simulink model "RobotModel8"  (R2025b)
settings: Solver=VariableStepAuto  StartTime=0.0  StopTime=150  RelTol=0.01  AbsTol=0.01  EnableMultiTasking=on
values from neighbouring files (symbols this model uses):
  waypoints = [R*cos(theta)+5, R*sin(theta)]    [init_waypoints.m]
undefined symbols (not defined in the file or in its folder): X, Y, Z
libraries: sm_lib x71, nesl_utility x45, slpidlib x2, robotalgslib x1, sharedtransform x1
(part 4 of 5)

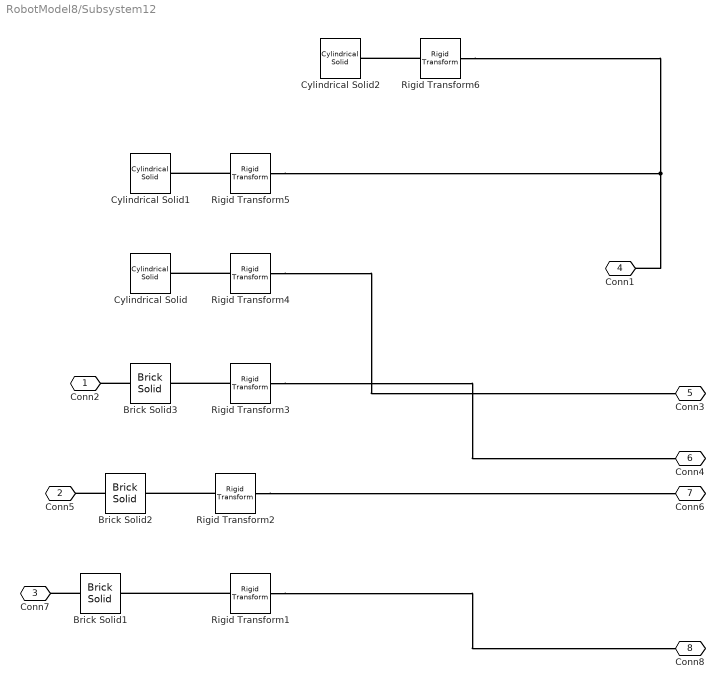
== system RobotModel8/Subsystem12 ==
  Brick Solid1 : sm_lib/Body Elements/Brick Solid  BrickDimensions=[14.5 7.3 2]  BrickDimensionsUnits=m  ExportEntireGeometry=on  InertiaType=CalculateFromGeometry  BasedOnType=Density  Density=1000  DensityUnits=kg/m^3  Mass=1  MassUnits=kg  CenterOfMass=[0 0 0]  CenterOfMassUnits=m  MomentsOfInertia=[1 1 1]  MomentsOfInertiaUnits=kg*m^2  ProductsOfInertia=[0 0 0]  ProductsOfInertiaUnits=kg*m^2  GraphicType=FromGeometry  MarkerShape=Sphere  MarkerSize=10  GraphicVisPropType=SimpleVisualProperties  GraphicDiffuseColor=[0.3333 0.1882 0.007843]  GraphicOpacity=1  GraphicSpecularColor=[0.5 0.5 0.5 1.0]  GraphicAmbientColor=[0.15 0.15 0.15 1.0]  GraphicEmissiveColor=[0.0 0.0 0.0 1.0]  GraphicShininess=75  DoExposeReferenceFrame=on  SerializedFrames=<Frames/>
  Brick Solid2 : sm_lib/Body Elements/Brick Solid  BrickDimensions=[12.4 9.9 2]  BrickDimensionsUnits=m  ExportEntireGeometry=on  InertiaType=CalculateFromGeometry  BasedOnType=Density  Density=1000  DensityUnits=kg/m^3  Mass=1  MassUnits=kg  CenterOfMass=[0 0 0]  CenterOfMassUnits=m  MomentsOfInertia=[1 1 1]  MomentsOfInertiaUnits=kg*m^2  ProductsOfInertia=[0 0 0]  ProductsOfInertiaUnits=kg*m^2  GraphicType=FromGeometry  MarkerShape=Sphere  MarkerSize=10  GraphicVisPropType=SimpleVisualProperties  GraphicDiffuseColor=[0.3333 0.1882 0.007843]  GraphicOpacity=1  GraphicSpecularColor=[0.5 0.5 0.5 1.0]  GraphicAmbientColor=[0.15 0.15 0.15 1.0]  GraphicEmissiveColor=[0.0 0.0 0.0 1.0]  GraphicShininess=75  DoExposeReferenceFrame=on  SerializedFrames=<Frames/>
  Brick Solid3 : sm_lib/Body Elements/Brick Solid  BrickDimensions=[10 10 2]  BrickDimensionsUnits=m  ExportEntireGeometry=on  InertiaType=CalculateFromGeometry  BasedOnType=Density  Density=1000  DensityUnits=kg/m^3  Mass=1  MassUnits=kg  CenterOfMass=[0 0 0]  CenterOfMassUnits=m  MomentsOfInertia=[1 1 1]  MomentsOfInertiaUnits=kg*m^2  ProductsOfInertia=[0 0 0]  ProductsOfInertiaUnits=kg*m^2  GraphicType=FromGeometry  MarkerShape=Sphere  MarkerSize=10  GraphicVisPropType=SimpleVisualProperties  GraphicDiffuseColor=[0.3333 0.1882 0.007843]  GraphicOpacity=1  GraphicSpecularColor=[0.5 0.5 0.5 1.0]  GraphicAmbientColor=[0.15 0.15 0.15 1.0]  GraphicEmissiveColor=[0.0 0.0 0.0 1.0]  GraphicShininess=75  DoExposeReferenceFrame=on  SerializedFrames=<Frames/>
  Cylindrical Solid : sm_lib/Body Elements/Cylindrical Solid  CylinderRadius=6  CylinderRadiusUnits=m  CylinderLength=2  CylinderLengthUnits=m  ExportEntireGeometry=off  InertiaType=CalculateFromGeometry  BasedOnType=Density  Density=1000  DensityUnits=kg/m^3  Mass=1  MassUnits=kg  CenterOfMass=[0 0 0]  CenterOfMassUnits=m  MomentsOfInertia=[1 1 1]  MomentsOfInertiaUnits=kg*m^2  ProductsOfInertia=[0 0 0]  ProductsOfInertiaUnits=kg*m^2  GraphicType=FromGeometry  MarkerShape=Sphere  MarkerSize=10  GraphicVisPropType=SimpleVisualProperties  GraphicDiffuseColor=[0.3333 0.1882 0.007843]  GraphicOpacity=1  GraphicSpecularColor=[0.5 0.5 0.5 1.0]  GraphicAmbientColor=[0.15 0.15 0.15 1.0]  GraphicEmissiveColor=[0.0 0.0 0.0 1.0]  GraphicShininess=75  DoExposeReferenceFrame=on  SerializedFrames=<Frames/>
  Cylindrical Solid1 : sm_lib/Body Elements/Cylindrical Solid  CylinderRadius=5  CylinderRadiusUnits=m  CylinderLength=2  CylinderLengthUnits=m  ExportEntireGeometry=off  InertiaType=CalculateFromGeometry  BasedOnType=Density  Density=1000  DensityUnits=kg/m^3  Mass=1  MassUnits=kg  CenterOfMass=[0 0 0]  CenterOfMassUnits=m  MomentsOfInertia=[1 1 1]  MomentsOfInertiaUnits=kg*m^2  ProductsOfInertia=[0 0 0]  ProductsOfInertiaUnits=kg*m^2  GraphicType=FromGeometry  MarkerShape=Sphere  MarkerSize=10  GraphicVisPropType=SimpleVisualProperties  GraphicDiffuseColor=[0.3333 0.1882 0.007843]  GraphicOpacity=1  GraphicSpecularColor=[0.5 0.5 0.5 1.0]  GraphicAmbientColor=[0.15 0.15 0.15 1.0]  GraphicEmissiveColor=[0.0 0.0 0.0 1.0]  GraphicShininess=75  DoExposeReferenceFrame=on  SerializedFrames=<Frames/>
  Cylindrical Solid2 : sm_lib/Body Elements/Cylindrical Solid  CylinderRadius=5  CylinderRadiusUnits=m  CylinderLength=2  CylinderLengthUnits=m  ExportEntireGeometry=off  InertiaType=CalculateFromGeometry  BasedOnType=Density  Density=1000  DensityUnits=kg/m^3  Mass=1  MassUnits=kg  CenterOfMass=[0 0 0]  CenterOfMassUnits=m  MomentsOfInertia=[1 1 1]  MomentsOfInertiaUnits=kg*m^2  ProductsOfInertia=[0 0 0]  ProductsOfInertiaUnits=kg*m^2  GraphicType=FromGeometry  MarkerShape=Sphere  MarkerSize=10  GraphicVisPropType=SimpleVisualProperties  GraphicDiffuseColor=[0.3333 0.1882 0.007843]  GraphicOpacity=1  GraphicSpecularColor=[0.5 0.5 0.5 1.0]  GraphicAmbientColor=[0.15 0.15 0.15 1.0]  GraphicEmissiveColor=[0.0 0.0 0.0 1.0]  GraphicShininess=75  DoExposeReferenceFrame=on  SerializedFrames=<Frames/>
  Rigid Transform1 : sm_lib/Frames and Transforms/Rigid Transform  RotationMethod=None  FollAlignAxisA=+X  BaseAlignAxisA=+Y  FollAlignAxisB=+Y  BaseAlignAxisB=+Z  RotationStandardAxis=+Z  RotationAngle=90  RotationAngleUnits=deg  RotationArbitraryAxis=[0 0 1]  RotationSequenceAxes=FollowerAxes  RotationSequence=XYX  RotationSequenceAngles=[0 0 0]  RotationSequenceAnglesUnits=deg  RotationMatrix=[1 0 0;0 1 0;0 0 1]  Quaternion=[1 0 0 0]  TranslationMethod=Cartesian  TranslationCartesianOffset=[-15 -13.75 -1]  TranslationCartesianOffsetUnits=m  TranslationStandardAxis=+Z  TranslationStandardOffset=0  TranslationStandardOffsetUnits=m  TranslationROffset=0  TranslationROffsetUnits=m  TranslationThetaOffset=0  TranslationThetaOffsetUnits=deg  TranslationZOffset=0  TranslationZOffsetUnits=m
  Rigid Transform2 : sm_lib/Frames and Transforms/Rigid Transform  RotationMethod=None  FollAlignAxisA=+X  BaseAlignAxisA=+Y  FollAlignAxisB=+Y  BaseAlignAxisB=+Z  RotationStandardAxis=+Z  RotationAngle=90  RotationAngleUnits=deg  RotationArbitraryAxis=[0 0 1]  RotationSequenceAxes=FollowerAxes  RotationSequence=XYX  RotationSequenceAngles=[0 0 0]  RotationSequenceAnglesUnits=deg  RotationMatrix=[1 0 0;0 1 0;0 0 1]  Quaternion=[1 0 0 0]  TranslationMethod=Cartesian  TranslationCartesianOffset=[-21 -32.5 -1]  TranslationCartesianOffsetUnits=m  TranslationStandardAxis=+Z  TranslationStandardOffset=0  TranslationStandardOffsetUnits=m  TranslationROffset=0  TranslationROffsetUnits=m  TranslationThetaOffset=0  TranslationThetaOffsetUnits=deg  TranslationZOffset=0  TranslationZOffsetUnits=m
  Rigid Transform3 : sm_lib/Frames and Transforms/Rigid Transform  RotationMethod=None  FollAlignAxisA=+X  BaseAlignAxisA=+Y  FollAlignAxisB=+Y  BaseAlignAxisB=+Z  RotationStandardAxis=+Z  RotationAngle=90  RotationAngleUnits=deg  RotationArbitraryAxis=[0 0 1]  RotationSequenceAxes=FollowerAxes  RotationSequence=XYX  RotationSequenceAngles=[0 0 0]  RotationSequenceAnglesUnits=deg  RotationMatrix=[1 0 0;0 1 0;0 0 1]  Quaternion=[1 0 0 0]  TranslationMethod=Cartesian  TranslationCartesianOffset=[-37.5 -15 -1]  TranslationCartesianOffsetUnits=m  TranslationStandardAxis=+Z  TranslationStandardOffset=0  TranslationStandardOffsetUnits=m  TranslationROffset=0  TranslationROffsetUnits=m  TranslationThetaOffset=0  TranslationThetaOffsetUnits=deg  TranslationZOffset=0  TranslationZOffsetUnits=m
  Rigid Transform4 : sm_lib/Frames and Transforms/Rigid Transform  RotationMethod=None  FollAlignAxisA=+X  BaseAlignAxisA=+Y  FollAlignAxisB=+Y  BaseAlignAxisB=+Z  RotationStandardAxis=+Z  RotationAngle=90  RotationAngleUnits=deg  RotationArbitraryAxis=[0 0 1]  RotationSequenceAxes=FollowerAxes  RotationSequence=XYX  RotationSequenceAngles=[0 0 0]  RotationSequenceAnglesUnits=deg  RotationMatrix=[1 0 0;0 1 0;0 0 1]  Quaternion=[1 0 0 0]  TranslationMethod=Cartesian  TranslationCartesianOffset=[-15 -37.5 -1]  TranslationCartesianOffsetUnits=m  TranslationStandardAxis=+Z  TranslationStandardOffset=0  TranslationStandardOffsetUnits=m  TranslationROffset=0  TranslationROffsetUnits=m  TranslationThetaOffset=0  TranslationThetaOffsetUnits=deg  TranslationZOffset=0  TranslationZOffsetUnits=m
  Rigid Transform5 : sm_lib/Frames and Transforms/Rigid Transform  RotationMethod=None  FollAlignAxisA=+X  BaseAlignAxisA=+Y  FollAlignAxisB=+Y  BaseAlignAxisB=+Z  RotationStandardAxis=+Z  RotationAngle=90  RotationAngleUnits=deg  RotationArbitraryAxis=[0 0 1]  RotationSequenceAxes=FollowerAxes  RotationSequence=XYX  RotationSequenceAngles=[0 0 0]  RotationSequenceAnglesUnits=deg  RotationMatrix=[1 0 0;0 1 0;0 0 1]  Quaternion=[1 0 0 0]  TranslationMethod=Cartesian  TranslationCartesianOffset=[-35 -30 -1]  TranslationCartesianOffsetUnits=m  TranslationStandardAxis=+Z  TranslationStandardOffset=0  TranslationStandardOffsetUnits=m  TranslationROffset=0  TranslationROffsetUnits=m  TranslationThetaOffset=0  TranslationThetaOffsetUnits=deg  TranslationZOffset=0  TranslationZOffsetUnits=m
  Rigid Transform6 : sm_lib/Frames and Transforms/Rigid Transform  RotationMethod=None  FollAlignAxisA=+X  BaseAlignAxisA=+Y  FollAlignAxisB=+Y  BaseAlignAxisB=+Z  RotationStandardAxis=+Z  RotationAngle=90  RotationAngleUnits=deg  RotationArbitraryAxis=[0 0 1]  RotationSequenceAxes=FollowerAxes  RotationSequence=XYX  RotationSequenceAngles=[0 0 0]  RotationSequenceAnglesUnits=deg  RotationMatrix=[1 0 0;0 1 0;0 0 1]  Quaternion=[1 0 0 0]  TranslationMethod=Cartesian  TranslationCartesianOffset=[-25 -12.5 -1]  TranslationCartesianOffsetUnits=m  TranslationStandardAxis=+Z  TranslationStandardOffset=0  TranslationStandardOffsetUnits=m  TranslationROffset=0  TranslationROffsetUnits=m  TranslationThetaOffset=0  TranslationThetaOffsetUnits=deg  TranslationZOffset=0  TranslationZOffsetUnits=m
  Conn2 : PMIOPort  Side=Left
  Conn5 : PMIOPort  Port=2  Side=Left
  Conn7 : PMIOPort  Port=3  Side=Left
  Conn1 : PMIOPort  Port=4  Side=Right
  Conn3 : PMIOPort  Port=5  Side=Right
  Conn4 : PMIOPort  Port=6  Side=Right
  Conn6 : PMIOPort  Port=7  Side=Right
  Conn8 : PMIOPort  Port=8  Side=Right
  connections:
  Rigid Transform1/LConn1 -- Brick Solid1/RConn1
  Rigid Transform5/LConn1 -- Cylindrical Solid1/RConn1
  Rigid Transform3/LConn1 -- Brick Solid3/RConn1
  Rigid Transform5/RConn1 -- Conn1/RConn1 -- Rigid Transform6/RConn1
  Brick Solid2/LConn1 -- Conn5/RConn1
  Rigid Transform1/RConn1 -- Conn8/RConn1
  Rigid Transform4/RConn1 -- Conn3/RConn1
  Rigid Transform6/LConn1 -- Cylindrical Solid2/RConn1
  Rigid Transform4/LConn1 -- Cylindrical Solid/RConn1
  Rigid Transform2/LConn1 -- Brick Solid2/RConn1
  Rigid Transform3/RConn1 -- Conn4/RConn1
  Rigid Transform2/RConn1 -- Conn6/RConn1
  Brick Solid1/LConn1 -- Conn7/RConn1
  Brick Solid3/LConn1 -- Conn2/RConn1

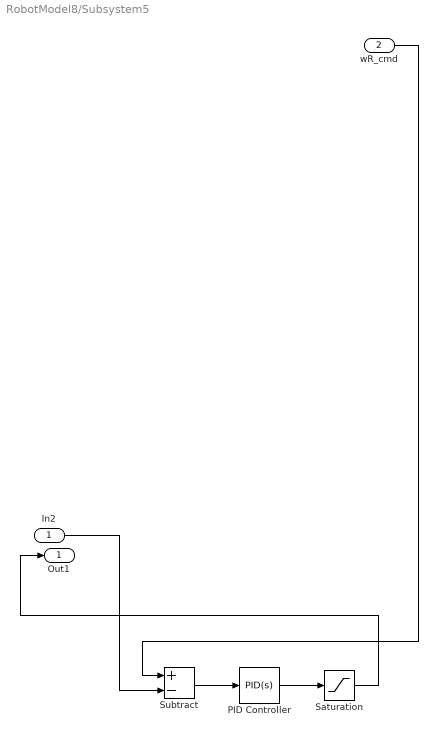
== system RobotModel8/Subsystem5 ==
  In2 : Inport
  wR_cmd : Inport  Port=2
  PID Controller : slpidlib/PID Controller  Controller=PID  Form=Parallel  TimeDomain=Continuous-time  UseExternalTs=off  SampleTime=-1  IntegratorMethod=Forward Euler  FilterMethod=Forward Euler  ControllerParametersSource=internal  P=5  I=0  UseKiTs=off  D=0  UseExternalDerivativeSource=off  N=100  UseFilter=on  TunerSelectOption=Transfer Function Based (PID Tuner App)  InitialConditionSource=internal  InitialConditionForIntegrator=0  InitialConditionForFilter=0  DifferentiatorICPrevScaledInput=0  ExternalReset=none  TrackingMode=off  Kt=1  LimitOutput=off  SatLimitsSource=internal  UpperSaturationLimit=inf  LowerSaturationLimit=-inf  LinearizeAsGain=on  AntiWindupMode=none  Kb=1  LimitIntegrator=off  UpperIntegratorSaturationLimit=inf  LowerIntegratorSaturationLimit=-inf  POutMin=[]  POutMax=[]  IOutMin=[]  IOutMax=[]  DOutMin=[]  DOutMax=[]  NOutMin=[]  NOutMax=[]  SumOutMin=[]  SumOutMax=[]  SaturationOutMin=[]  SaturationOutMax=[]  PParamMin=[]  PParamMax=[]  IParamMin=[]  IParamMax=[]  DParamMin=[]  DParamMax=[]  NParamMin=[]  NParamMax=[]  KbParamMin=[]  KbParamMax=[]  KtParamMin=[]  KtParamMax=[]  KbOutMin=[]  KbOutMax=[]  KtOutMin=[]  KtOutMax=[]  IntegratorOutMin=[]  IntegratorOutMax=[]  FilterOutMin=[]  FilterOutMax=[]  SumI1OutMin=[]  SumI1OutMax=[]  SumI2OutMin=[]  SumI2OutMax=[]  SumI3OutMin=[]  SumI3OutMax=[]  SumI4OutMin=[]  SumI4OutMax=[]  SumDOutMin=[]  SumDOutMax=[]  DifferentiatorOutMin=[]  DifferentiatorOutMax=[]  FilterDiffOutCoefMin=[]  FilterDiffOutCoefMax=[]  ReciprocalOutMin=[]  ReciprocalOutMax=[]  SumDenOutMin=[]  SumDenOutMax=[]  SumNumOutMin=[]  SumNumOutMax=[]  DivideOutMin=[]  DivideOutMax=[]  UdiffTsProdOutMin=[]  UdiffTsProdOutMax=[]  NTsProdOutMin=[]  NTsProdOutMax=[]  UintegralTsProdOutMin=[]  UintegralTsProdOutMax=[]  UngainTsProdOutMin=[]  UngainTsProdOutMax=[]  ClampingZeroOutDataTypeStr=Inherit: Inherit via back propagation  ClampingZeroOutMin=[]  ClampingZeroOutMax=[]  FilterDenConstantOutDataTypeStr=Inherit: Inherit via back propagation  FilterDenConstantOutMin=[]  FilterDenConstantOutMax=[]  PCopyOutDataTypeStr=Inherit: Inherit via back propagation  PCopyOutMin=[]  PCopyOutMax=[]  NCopyOutDataTypeStr=Inherit: Inherit via back propagation  NCopyOutMin=[]  NCopyOutMax=[]  IntegratorContinuousStateAttributes=''  IntegratorStateMustResolveToSignalObject=off  IntegratorRTWStateStorageClass=Auto  FilterContinuousStateAttributes=''  FilterStateMustResolveToSignalObject=off  FilterRTWStateStorageClass=Auto  ParallelPVariant=InternalParameters  IdealPVariant=Disabled  IVariant=InternalParameters  DVariant=InternalParameters  IntegratorVariant=Continuous  SatVariant=Disabled  AWVariant=Passthrough  PCopyVariant=Disabled  TRVariant=Disabled  FdbkBlocksVariant=Forward  IdealPFdbkVariant=Disabled  SatFdbkVariant=Disabled  DerivativeFilterVariant=ContFilter  NVariant=InternalParameters  NCopyVariant=Disabled  FilterICVariant=InternalICsFilter  IntegratorICVariant=InternalICs  ExternalResetVariant=Disabled  TRSumVariant=Passthrough  SumFdbkVariant=Disabled  SumVariant=Sum_PID  TsampFilterVariant=InternalTs  TsampNgainVariant=Passthrough  TsampIntegralVariant=Disabled_SignalSpec  ExternalSaturationOutDataTypeStr=Inherit: Same as second input  DerivativeSourceVariant=ErrorSignal  PreIntVariant=InternalPreInt
  Saturation : Saturate  UpperLimit=5  LowerLimit=-5
  Subtract : Sum  Inputs=+-
  Out1 : Outport
  wires:
  In2/1 -> Subtract/2
  Subtract/1 -> PID Controller/1
  Saturation/1 -> Out1/1
  PID Controller/1 -> Saturation/1
  wR_cmd/1 -> Subtract/1

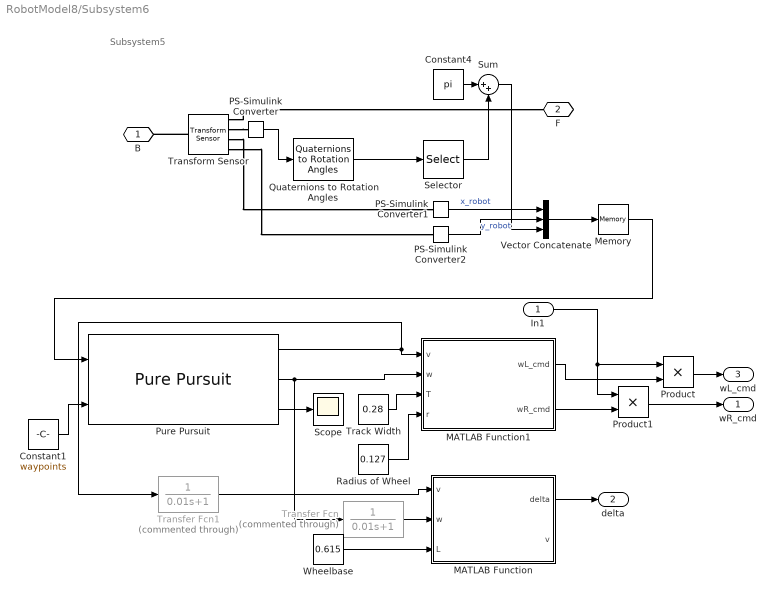
== system RobotModel8/Subsystem6 ==
  note: Subsystem5
  In1 : Inport
  Constant1 : Constant  Value=waypoints
  Constant4 : Constant  Value=pi
  MATLAB Function : MATLAB Function  TreatAsAtomicUnit=on
  MATLAB Function1 : MATLAB Function  TreatAsAtomicUnit=on
  Memory : Memory
  PS-Simulink Converter : nesl_utility/PS-Simulink Converter  PhysicalDomain=network_engine_domain  SubClassName=ps_output  LeftPortType=input  RightPortType=output  PseudoPeriodic=off  Frequencies=[]  VectorFormat=inherit  Unit=inherit  AffineConversion=off
  PS-Simulink Converter1 : nesl_utility/PS-Simulink Converter  PhysicalDomain=network_engine_domain  SubClassName=ps_output  LeftPortType=input  RightPortType=output  PseudoPeriodic=off  Frequencies=[]  VectorFormat=inherit  Unit=inherit  AffineConversion=off
  PS-Simulink Converter2 : nesl_utility/PS-Simulink Converter  PhysicalDomain=network_engine_domain  SubClassName=ps_output  LeftPortType=input  RightPortType=output  PseudoPeriodic=off  Frequencies=[]  VectorFormat=inherit  Unit=inherit  AffineConversion=off
  Product : Product
  Product1 : Product
  Pure Pursuit : robotalgslib/Pure Pursuit  DesiredLinearVelocityPort=off  DesiredLinearVelocity=0.7  MaxAngularVelocity=0.8  LookaheadDistancePort=off  LookaheadDistance=0.6  TargetDirPort=on  SimulateUsing=Code generation
      settings: LibrarySourceBlock=navlib/Control Algorithms/Pure Pursuit
  Quaternions to Rotation Angles : sharedtransform/Quaternions to Rotation Angles  rotationOrder=ZYX  aMode=aMode
  Radius of Wheel : Constant  Value=0.127
  Scope : Scope
      settings: ActiveDisplayYMinimum=-49.938512022124293  ActiveDisplayYMaximum=229.50278461957694
  Selector : Selector  InputPortWidth=3  IndexOptions=Index vector (dialog)  Indices=[1]  OutputSizes=1
  Sum : Sum  Inputs=|++
  Track Width : Constant  Value=0.28
  Transfer Fcn : TransferFcn  Commented=through  Denominator=[0.01 1]
  Transfer Fcn1 : TransferFcn  Commented=through  Denominator=[0.01 1]
  Transform Sensor : sm_lib/Frames and Transforms/Transform Sensor  MeasurementFrame=World  RotationSequence=XYX  SenseAngle=off  SenseAxis=off  SenseQ=on  SenseR=off  SenseRotationSequence=off  SenseOmegaX=off  SenseOmegaY=off  SenseOmegaZ=off  SenseOmega=off  SenseQDot=off  SenseRDot=off  SenseRotationSequenceDot=off  SenseAlphaX=off  SenseAlphaY=off  SenseAlphaZ=off  SenseAlpha=off  SenseQDDot=off  SenseRDDot=off  SenseX=on  SenseY=on  SenseZ=off  SenseXYZ=off  SenseRad=off  SenseAzim=off  SenseDist=off  SenseInc=off  SenseXDot=off  SenseYDot=off  SenseZDot=off  SenseXYZDot=off  SenseRadDot=off  SenseAzimDot=off  SenseDistDot=off  SenseIncDot=off  SenseXDDot=off  SenseYDDot=off  SenseZDDot=off  SenseXYZDDot=off  SenseRadDDot=off  SenseAzimDDot=off  SenseDistDDot=off  SenseIncDDot=off
  Vector Concatenate : Concatenate  NumInputs=3
  Wheelbase : Constant  Value=0.615
  B : PMIOPort  Side=Left
  F : PMIOPort  Port=2  Side=Right
  wR_cmd : Outport
  delta : Outport  Port=2
  wL_cmd : Outport  Port=3
  wires:
  Pure Pursuit/2 -> MATLAB Function1/2(w), Transfer Fcn/1
  Transfer Fcn1/1 -> MATLAB Function/1("v ")
  Transfer Fcn/1 -> MATLAB Function/2(w)
  Constant1/1 -> Pure Pursuit/2
  Radius of Wheel/1 -> MATLAB Function1/4(r)
  Track Width/1 -> MATLAB Function1/3(T)
  Wheelbase/1 -> MATLAB Function/3(L)
  Pure Pursuit/1 -> MATLAB Function1/1(v), Transfer Fcn1/1
  Pure Pursuit/3 -> Scope/1
  Memory/1 -> Pure Pursuit/1
  In1/1 -> Product/1, Product1/1
  MATLAB Function1/1(wL_cmd) -> Product/2
  Product/1 -> wL_cmd/1
  MATLAB Function1/2(wR_cmd) -> Product1/2
  Product1/1 -> wR_cmd/1
  MATLAB Function/1(delta) -> delta/1
  Sum/1 -> Vector Concatenate/3
  Selector/1 -> Sum/2
  Constant4/1 -> Sum/1
  PS-Simulink Converter2/1 -> Vector Concatenate/2  "y_robot"
  PS-Simulink Converter1/1 -> Vector Concatenate/1  "x_robot"
  Vector Concatenate/1 -> Memory/1
  PS-Simulink Converter/1 -> Quaternions to Rotation Angles/1
  Quaternions to Rotation Angles/1 -> Selector/1
  connections:
  Transform Sensor/RConn1 -- F/RConn1
  Transform Sensor/LConn1 -- B/RConn1
  Transform Sensor/RConn3 -- PS-Simulink Converter1/LConn1
  Transform Sensor/RConn2 -- PS-Simulink Converter/LConn1
  Transform Sensor/RConn4 -- PS-Simulink Converter2/LConn1

== system RobotModel8/Subsystem7 ==
  wL_cmd : Inport
  In2 : Inport  Port=2
  PID Controller : slpidlib/PID Controller  Controller=PID  Form=Parallel  TimeDomain=Continuous-time  UseExternalTs=off  SampleTime=-1  IntegratorMethod=Forward Euler  FilterMethod=Forward Euler  ControllerParametersSource=internal  P=5  I=0  UseKiTs=off  D=0  UseExternalDerivativeSource=off  N=100  UseFilter=on  TunerSelectOption=Transfer Function Based (PID Tuner App)  InitialConditionSource=internal  InitialConditionForIntegrator=0  InitialConditionForFilter=0  DifferentiatorICPrevScaledInput=0  ExternalReset=none  TrackingMode=off  Kt=1  LimitOutput=off  SatLimitsSource=internal  UpperSaturationLimit=inf  LowerSaturationLimit=-inf  LinearizeAsGain=on  AntiWindupMode=none  Kb=1  LimitIntegrator=off  UpperIntegratorSaturationLimit=inf  LowerIntegratorSaturationLimit=-inf  POutMin=[]  POutMax=[]  IOutMin=[]  IOutMax=[]  DOutMin=[]  DOutMax=[]  NOutMin=[]  NOutMax=[]  SumOutMin=[]  SumOutMax=[]  SaturationOutMin=[]  SaturationOutMax=[]  PParamMin=[]  PParamMax=[]  IParamMin=[]  IParamMax=[]  DParamMin=[]  DParamMax=[]  NParamMin=[]  NParamMax=[]  KbParamMin=[]  KbParamMax=[]  KtParamMin=[]  KtParamMax=[]  KbOutMin=[]  KbOutMax=[]  KtOutMin=[]  KtOutMax=[]  IntegratorOutMin=[]  IntegratorOutMax=[]  FilterOutMin=[]  FilterOutMax=[]  SumI1OutMin=[]  SumI1OutMax=[]  SumI2OutMin=[]  SumI2OutMax=[]  SumI3OutMin=[]  SumI3OutMax=[]  SumI4OutMin=[]  SumI4OutMax=[]  SumDOutMin=[]  SumDOutMax=[]  DifferentiatorOutMin=[]  DifferentiatorOutMax=[]  FilterDiffOutCoefMin=[]  FilterDiffOutCoefMax=[]  ReciprocalOutMin=[]  ReciprocalOutMax=[]  SumDenOutMin=[]  SumDenOutMax=[]  SumNumOutMin=[]  SumNumOutMax=[]  DivideOutMin=[]  DivideOutMax=[]  UdiffTsProdOutMin=[]  UdiffTsProdOutMax=[]  NTsProdOutMin=[]  NTsProdOutMax=[]  UintegralTsProdOutMin=[]  UintegralTsProdOutMax=[]  UngainTsProdOutMin=[]  UngainTsProdOutMax=[]  ClampingZeroOutDataTypeStr=Inherit: Inherit via back propagation  ClampingZeroOutMin=[]  ClampingZeroOutMax=[]  FilterDenConstantOutDataTypeStr=Inherit: Inherit via back propagation  FilterDenConstantOutMin=[]  FilterDenConstantOutMax=[]  PCopyOutDataTypeStr=Inherit: Inherit via back propagation  PCopyOutMin=[]  PCopyOutMax=[]  NCopyOutDataTypeStr=Inherit: Inherit via back propagation  NCopyOutMin=[]  NCopyOutMax=[]  IntegratorContinuousStateAttributes=''  IntegratorStateMustResolveToSignalObject=off  IntegratorRTWStateStorageClass=Auto  FilterContinuousStateAttributes=''  FilterStateMustResolveToSignalObject=off  FilterRTWStateStorageClass=Auto  ParallelPVariant=InternalParameters  IdealPVariant=Disabled  IVariant=InternalParameters  DVariant=InternalParameters  IntegratorVariant=Continuous  SatVariant=Disabled  AWVariant=Passthrough  PCopyVariant=Disabled  TRVariant=Disabled  FdbkBlocksVariant=Forward  IdealPFdbkVariant=Disabled  SatFdbkVariant=Disabled  DerivativeFilterVariant=ContFilter  NVariant=InternalParameters  NCopyVariant=Disabled  FilterICVariant=InternalICsFilter  IntegratorICVariant=InternalICs  ExternalResetVariant=Disabled  TRSumVariant=Passthrough  SumFdbkVariant=Disabled  SumVariant=Sum_PID  TsampFilterVariant=InternalTs  TsampNgainVariant=Passthrough  TsampIntegralVariant=Disabled_SignalSpec  ExternalSaturationOutDataTypeStr=Inherit: Same as second input  DerivativeSourceVariant=ErrorSignal  PreIntVariant=InternalPreInt
  Saturation : Saturate  UpperLimit=5  LowerLimit=-5
  Subtract : Sum  Inputs=+-
  Out1 : Outport
  wires:
  In2/1 -> Subtract/2
  Subtract/1 -> PID Controller/1
  Saturation/1 -> Out1/1
  PID Controller/1 -> Saturation/1
  wL_cmd/1 -> Subtract/1

== matlab function RobotModel8/RL/MATLAB Function1 ==
  data: mode_cmd input; alpha input; tau output; q input; dq input; q_cmd input; is_locked output; q_ref output
function [tau, is_locked, q_ref] = LockJointPD(mode_cmd, alpha, q, dq, q_cmd)
%#codegen
% mode_cmd: 0=Walk (track q_cmd), 1=Wheeled (lock current angle)
% alpha   : [0,1] smoothing factor (TransferFcn output), 0=fully walking, 1=fully locked
% q,dq    : joint angle/angular velocity
% q_cmd   : walk/stand target angle (radians)
Kp = 1200.0;   % Starting value, tune per joint
Kd =   20.0;
tau_lim = 300.0;
m = uint8(mode_cmd ~= 0);     % Standardize to uint8(0/1)
a = double(alpha);
persistent q_hold last_mode
if isempty(q_hold),    q_hold    = q;        end   % double
if isempty(last_mode), last_mode = uint8(0); end   % uint8
% Rising edge: 0->1, latch current angle
if (last_mode == uint8(0)) && (m ~= uint8(0))
    q_hold = q;
end
last_mode = m;
% Reference angle: interpolate between "hold angle" and "target angle"
q_ref  = a*q_hold + (1-a)*q_cmd;
dq_ref = 0.0;
% PD
tau = Kp*(q_ref - q) + Kd*(dq_ref - dq);
% Saturation
tau = max(min(tau, tau_lim), -tau_lim);
% Debug flag: is leg lock dominant
is_locked = (a > 0.5);     % Can also output m==1
end

== matlab function RobotModel8/Subsystem6/MATLAB Function1 ==
  data: v input; wL_cmd output; w input; T input; r input; wR_cmd output
function [wL_cmd, wR_cmd] = wheelSpeedCmd(v, w, T, r)
% v: linear velocity [m/s]
% w: 航向角速度 [rad/s]
% T: 后轮距 [m]
% r: 车轮半径 [m]

vL = v - 0.5*T*w;
vR = v + 0.5*T*w;

wL_cmd = vL / r;
wR_cmd = vR / r;
end

== matlab function RobotModel8/Subsystem6/MATLAB Function ==
  data: v input; delta output; w input; L input; v output
function [delta, v] = Diff2Ackermann(v, w, L)
% input: 
%   v - Linear velocity (m/s)
%   w - Angular velocity (rad/s)
%   L - Wheelbase (m)
%
% output:
%   delta - front wheel rotation angel (rad)
%   v     -  velocity(m/s)
if abs(v) < 1e-3
    delta = 0;
else
    delta = atan(L * w / v);   % pure pursuit function
end

== matlab function RobotModel8/RR_climb/MATLAB Function ==
  data: t input; q output; mode_cmd input
function q = knee_FL_motion(t, mode_cmd)
%#codegen

Tsw = 102;   % 切换时间

% ------- 轮式模式：锁住，腿不动 -------
if (mode_cmd == 1) || (t < Tsw)
    q = 0;          % 回到原位（站立角）
    return;
end

% ------- 腿式模式：先蹲再站 -------
tau = t - Tsw;      % 本地时间

% 对应髋关节的三个阶段：T1 蹲下，T2 保持，T3 站起
T1 = 3;    % 蹲下用时
T2 = 15;    % 低姿态保持时间
T3 = 3;    % 站起用时

% 膝关节的站立角和蹲下角
q_stand = 0;                % 站立时膝盖角（回原位就是这个）
q_squat = -deg2rad(70);      % 蹲下时膝盖最大弯曲

% --- 段1：从站立 -> 蹲下 ---
if tau < T1
    u = tau / T1;                           % 0→1
    q = (1-u)*q_stand + u*q_squat;

% --- 段2：保持蹲下姿态 ---
elseif tau < T1 + T2
    q = q_squat;

% --- 段3：从蹲下 -> 回到原位 ---
elseif tau < T1 + T2 + T3
    u = (tau - (T1 + T2)) / T3;
    q = (1-u)*q_squat + u*q_stand;

% --- 结束后一直保持原位 ---
else
    q = q_stand;
end
end

== matlab function RobotModel8/RL/MATLAB Function2 ==
  data: t input; w output
function w = wheel_speed(t)
%#codegen

Tsw  = 105;   % 初次开始加速时间
Tacc = 2;     % 加速时间
V    = 100;   % 力矩幅值
Tdec_start = 125;   % 开始减速
Tdec = 3;           % 减速时间

% --------------------
% 阶段 1：未开始
% --------------------
if t < Tsw
    w = 0;

% --------------------
% 阶段 2：线性加速 0→V
% --------------------
elseif t < Tsw + Tacc
    u = (t - Tsw) / Tacc;
    w = u * V;

% --------------------
% 阶段 3：保持 V
% --------------------
elseif t < Tdec_start
    w = V;

% --------------------
% 阶段 4：线性减速 V→0
% --------------------
elseif t < Tdec_start + Tdec
    u = (t - Tdec_start) / Tdec;  % 0→1
    w = V * (1 - u);

else
    w = 0;
end
end

== matlab function RobotModel8/FR_climb/MATLAB Function2 ==
  data: t input; q output; mode_cmd input
function q = knee_FL_motion(t, mode_cmd)
%#codegen

Tsw = 102;   % 切换时间

% ------- 轮式模式：锁住，腿不动 -------
if (mode_cmd == 1) || (t < Tsw)
    q = 0;          % 回到原位（站立角）
    return;
end

% ------- 腿式模式：先蹲再站 -------
tau = t - Tsw;      % 本地时间

% 对应髋关节的三个阶段：T1 蹲下，T2 保持，T3 站起
T1 = 3;    % 蹲下用时
T2 = 15;    % 低姿态保持时间
T3 = 3;    % 站起用时

% 膝关节的站立角和蹲下角
q_stand = 0;                % 站立时膝盖角（回原位就是这个）
q_squat = -deg2rad(70);      % 蹲下时膝盖最大弯曲

% --- 段1：从站立 -> 蹲下 ---
if tau < T1
    u = tau / T1;                           % 0→1
    q = (1-u)*q_stand + u*q_squat;

% --- 段2：保持蹲下姿态 ---
elseif tau < T1 + T2
    q = q_squat;

% --- 段3：从蹲下 -> 回到原位 ---
elseif tau < T1 + T2 + T3
    u = (tau - (T1 + T2)) / T3;
    q = (1-u)*q_squat + u*q_stand;

% --- 结束后一直保持原位 ---
else
    q = q_stand;
end
end

== matlab function RobotModel8/RL_climb/MATLAB Function ==
  data: t input; q output; mode_cmd input
function q = knee_FL_motion(t, mode_cmd)
%#codegen

Tsw = 102;   % 切换时间

% ------- 轮式模式：锁住，腿不动 -------
if (mode_cmd == 1) || (t < Tsw)
    q = 0;          % 回到原位（站立角）
    return;
end

% ------- 腿式模式：先蹲再站 -------
tau = t - Tsw;      % 本地时间

% 对应髋关节的三个阶段：T1 蹲下，T2 保持，T3 站起
T1 = 3;    % 蹲下用时
T2 = 15;    % 低姿态保持时间
T3 = 3;    % 站起用时

% 膝关节的站立角和蹲下角
q_stand = 0;                % 站立时膝盖角（回原位就是这个）
q_squat = -deg2rad(70);      % 蹲下时膝盖最大弯曲

% --- 段1：从站立 -> 蹲下 ---
if tau < T1
    u = tau / T1;                           % 0→1
    q = (1-u)*q_stand + u*q_squat;

% --- 段2：保持蹲下姿态 ---
elseif tau < T1 + T2
    q = q_squat;

% --- 段3：从蹲下 -> 回到原位 ---
elseif tau < T1 + T2 + T3
    u = (tau - (T1 + T2)) / T3;
    q = (1-u)*q_squat + u*q_stand;

% --- 结束后一直保持原位 ---
else
    q = q_stand;
end
end

== matlab function RobotModel8/RR/MATLAB Function1 ==
  data: mode_cmd input; alpha input; tau output; q input; dq input; q_cmd input; is_locked output; q_ref output
function [tau, is_locked, q_ref] = LockJointPD(mode_cmd, alpha, q, dq, q_cmd)
%#codegen
% mode_cmd: 0=Walk (track q_cmd), 1=Wheeled (lock current angle)
% alpha   : [0,1] smoothing factor (TransferFcn output), 0=fully walking, 1=fully locked
% q,dq    : joint angle/angular velocity
% q_cmd   : walk/stand target angle (radians)
Kp = 1200.0;   % Starting value, tune per joint
Kd =   20.0;
tau_lim = 300.0;
m = uint8(mode_cmd ~= 0);     % Standardize to uint8(0/1)
a = double(alpha);
persistent q_hold last_mode
if isempty(q_hold),    q_hold    = q;        end   % double
if isempty(last_mode), last_mode = uint8(0); end   % uint8
% Rising edge: 0->1, latch current angle
if (last_mode == uint8(0)) && (m ~= uint8(0))
    q_hold = q;
end
last_mode = m;
% Reference angle: interpolate between "hold angle" and "target angle"
q_ref  = a*q_hold + (1-a)*q_cmd;
dq_ref = 0.0;
% PD
tau = Kp*(q_ref - q) + Kd*(dq_ref - dq);
% Saturation
tau = max(min(tau, tau_lim), -tau_lim);
% Debug flag: is leg lock dominant
is_locked = (a > 0.5);     % Can also output m==1
end

== matlab function RobotModel8/RL/MATLAB Function3 ==
  data: brake_en input; tau output; w input
function tau = BrakeTorque(brake_en, w)
%#codegen
% brake_en: 0=不刹车, 1=开始刹车
% w: 轮子角速度 (rad/s)，来自 Revolute Joint 的 Velocity 输出

Kb = 30.0;       % 阻尼系数，越大刹车越狠，可调
tau_max = 150.0; % 最大刹车扭矩限幅
w_eps = 0.05;    % 认为“已经停下”的速度阈值

if brake_en == 0
    tau = 0.0;     % 不刹车
    return;
end

% 速度很小就不再给力，避免抖动
if abs(w) < w_eps
    tau = 0.0;
else
    % 阻尼刹车：扭矩方向与角速度相反
    tau = -Kb * w;
end

% 扭矩限幅
if tau >  tau_max, tau =  tau_max; end
if tau < -tau_max, tau = -tau_max; end
end

== matlab function RobotModel8/FL/MATLAB Function2 ==
  data: t input; w output
function w = wheel_speed(t)
%#codegen

Tsw  = 105;   % 初次开始加速时间
Tacc = 2;     % 加速时间
V    = 100;   % 力矩幅值
Tdec_start = 125;   % 开始减速
Tdec = 3;           % 减速时间

% --------------------
% 阶段 1：未开始
% --------------------
if t < Tsw
    w = 0;

% --------------------
% 阶段 2：线性加速 0→V
% --------------------
elseif t < Tsw + Tacc
    u = (t - Tsw) / Tacc;
    w = u * V;

% --------------------
% 阶段 3：保持 V
% --------------------
elseif t < Tdec_start
    w = V;

% --------------------
% 阶段 4：线性减速 V→0
% --------------------
elseif t < Tdec_start + Tdec
    u = (t - Tdec_start) / Tdec;  % 0→1
    w = V * (1 - u);

else
    w = 0;
end
end

== matlab function RobotModel8/FL_climb/MATLAB Function2 ==
  data: t input; q output; mode_cmd input
function q = hip_FL_motion(t, mode_cmd)
%#codegen
% --- 左前腿 (Front Left) 髋关节 ---
% 策略：锁轮爬梯。先迈步，然后负责拉动身体前移。

T_squat_start = 102;
T_climb_start = 130;

% --- 阶段 0: 轮式/未开始 ---
if (mode_cmd == 1) || (t < T_squat_start); q = 0; return; end

% --- 阶段 1: 原地蹲起测试 (102s-130s) ---
if t < T_climb_start
    tau = t - T_squat_start;
    q_stand = 0; q_squat = deg2rad(35);
    T1 = 3; T2 = 15; T3 = 3;
    if tau < T1; u=tau/T1; q=(1-u)*q_stand+u*q_squat;
    elseif tau < T1+T2; q=q_squat;
    elseif tau < T1+T2+T3; u=(tau-(T1+T2))/T3; q=(1-u)*q_squat+u*q_stand;
    else; q=q_stand; end
    return;
end

% ==========================================
% 阶段 2: 锁轮爬台阶 (130s 开始)
% ==========================================
tau = t - T_climb_start;

% 参数 (小步幅)
    q_neutral = 0;
    q_fwd     = deg2rad(-5); % 往前伸
    
    % [130-132] 第一步：抬腿迈向前方
    if tau < 2.0
        u = tau / 2.0;
        q = (1-u)*q_neutral + u*q_fwd;
        
    % [132-134] 等待右前腿 (保持在前)
    elseif tau < 4.0
        q = q_fwd;
        
    % [134-138] 全身前移 (Body Shift)
    % 关键：此时腿是着地的，Hip从"前"转回"中立"，相当于把身体拉过去
    elseif tau < 8.0
        dt = tau - 4.0;
        u = dt / 4.0; % 给4秒慢慢拉，防止前轮打滑
        u_smooth = 0.5 * (1 - cos(u * pi));
        q = (1-u_smooth)*q_fwd + u_smooth*q_neutral;
        
    % [138+] 动作完成，保持中立
    else
        q = q_neutral;
    end
end

== matlab function RobotModel8/FL_climb/MATLAB Function1 ==
  data: t input; q output; mode_cmd input
function q = knee_FL_motion(t, mode_cmd)
%#codegen

Tsw = 102;   % 切换时间

% ------- 轮式模式：锁住，腿不动 -------
if (mode_cmd == 1) || (t < Tsw)
    q = 0;          % 回到原位（站立角）
    return;
end

% ------- 腿式模式：先蹲再站 -------
tau = t - Tsw;      % 本地时间

% 对应髋关节的三个阶段：T1 蹲下，T2 保持，T3 站起
T1 = 3;    % 蹲下用时
T2 = 15;    % 低姿态保持时间
T3 = 3;    % 站起用时

% 膝关节的站立角和蹲下角
q_stand = 0;                % 站立时膝盖角（回原位就是这个）
q_squat = -deg2rad(70);      % 蹲下时膝盖最大弯曲

% --- 段1：从站立 -> 蹲下 ---
if tau < T1
    u = tau / T1;                           % 0→1
    q = (1-u)*q_stand + u*q_squat;

% --- 段2：保持蹲下姿态 ---
elseif tau < T1 + T2
    q = q_squat;

% --- 段3：从蹲下 -> 回到原位 ---
elseif tau < T1 + T2 + T3
    u = (tau - (T1 + T2)) / T3;
    q = (1-u)*q_squat + u*q_stand;

% --- 结束后一直保持原位 ---
else
    q = q_stand;
end
end

== matlab function RobotModel8/FL_climb/MATLAB Function3 ==
  data: t input; q output; mode_cmd input
function q = knee_FL_motion(t, mode_cmd)
%#codegen
% --- 左前腿 (Front Left) 膝关节 ---

T_squat_start = 102;
T_climb_start = 130;

% --- 阶段 0 & 1 ---
if (mode_cmd == 1) || (t < T_squat_start); q = 0; return; end
if t < T_climb_start
    tau = t - T_squat_start;
    q_stand = 0; q_squat = -deg2rad(70);
    T1 = 3; T2 = 15; T3 = 3;
    if tau < T1; u=tau/T1; q=(1-u)*q_stand+u*q_squat;
    elseif tau < T1+T2; q=q_squat;
    elseif tau < T1+T2+T3; u=(tau-(T1+T2))/T3; q=(1-u)*q_squat+u*q_stand;
    else; q=q_stand; end
    return;
end

% ==========================================
% 阶段 2: 锁轮爬台阶 (130s 开始)
% ==========================================
 tau = t - T_climb_start;
% --- 膝盖参数 ---
q_stand = deg2rad(0); % 站立微屈
    q_lift  = deg2rad(-20); % 小幅度抬腿
    
    % [130-132] 抬腿迈步
    if tau < 2.0
        u = tau / 2.0;
        lift_scale = sin(u * pi); 
        q = q_stand + lift_scale * (q_lift - q_stand);
        
    % [132+] 之后一直踩在地上用力
    else
        q = q_stand;
    end
end

== matlab function RobotModel8/FR_climb/MATLAB Function3 ==
  data: t input; q output; mode_cmd input
function q = hip_FL_motion(t, mode_cmd)
%#codegen

Tsw = 102;

% 轮式阶段：髋关节锁在 0
if (mode_cmd == 1) || (t < Tsw)
    q = 0;          % 轮式时锁住髋关节
    return;
end

% 腿式阶段：开始做“先蹲后站”的动作
tau = t - Tsw;      % 本地时间，从切换时刻重新计

% 姿态角（单位：rad）
q_stand = 0;                  % 站立时髋角
q_squat = deg2rad(35);       % 蹲下时髋角（负是往上收腿）
% 你觉得不够矮可以再调大一点绝对值，比如 -45°

% 时间设置（和膝盖可以对应着来）
T1 = 3;    % 蹲下用时
T2 = 15;    % 低姿态保持时间
T3 = 3;    % 站起来用时
% 总时长 T1+T2+T3 之后保持站立

% --- 段1：从站立 -> 蹲下 ---
if tau < T1
    u = tau / T1;                      % 0→1
    q = (1-u)*q_stand + u*q_squat;

% --- 段2：保持蹲下姿态 ---
elseif tau < T1 + T2
    q = q_squat;

% --- 段3：从蹲下 -> 站回原位 ---
elseif tau < T1 + T2 + T3
    u = (tau - (T1 + T2)) / T3;
    q = (1-u)*q_squat + u*q_stand;

% --- 结束后：保持站立 ---
else
    q = q_stand;
end
end

== matlab function RobotModel8/RL_climb/MATLAB Function1 ==
  data: t input; mode_cmd input; q output
function q= hip_FL_motion(t, mode_cmd)
%#codegen

Tsw = 102;

% 轮式阶段：髋关节锁在 0
if (mode_cmd == 1) || (t < Tsw)
    q = 0;          % 轮式时锁住髋关节
    return;
end

% 腿式阶段：开始做“先蹲后站”的动作
tau = t - Tsw;      % 本地时间，从切换时刻重新计

% 姿态角（单位：rad）
q_stand = 0;                  % 站立时髋角
q_squat = deg2rad(35);       % 蹲下时髋角（负是往上收腿）
% 你觉得不够矮可以再调大一点绝对值，比如 -45°

% 时间设置（和膝盖可以对应着来）
T1 = 3;    % 蹲下用时
T2 = 15;    % 低姿态保持时间
T3 = 3;    % 站起来用时
% 总时长 T1+T2+T3 之后保持站立

% --- 段1：从站立 -> 蹲下 ---
if tau < T1
    u = tau / T1;                      % 0→1
    q = (1-u)*q_stand + u*q_squat;

% --- 段2：保持蹲下姿态 ---
elseif tau < T1 + T2
    q = q_squat;

% --- 段3：从蹲下 -> 站回原位 ---
elseif tau < T1 + T2 + T3
    u = (tau - (T1 + T2)) / T3;
    q = (1-u)*q_squat + u*q_stand;

% --- 结束后：保持站立 ---
else
    q = q_stand;
end
end

== matlab function RobotModel8/RR_climb/MATLAB Function1 ==
  data: t input; q output; mode_cmd input
function q = hip_FL_motion(t, mode_cmd)
%#codegen

Tsw = 102;

% 轮式阶段：髋关节锁在 0
if (mode_cmd == 1) || (t < Tsw)
    q = 0;          % 轮式时锁住髋关节
    return;
end

% 腿式阶段：开始做“先蹲后站”的动作
tau = t - Tsw;      % 本地时间，从切换时刻重新计

% 姿态角（单位：rad）
q_stand = 0;                  % 站立时髋角
q_squat = deg2rad(35);       % 蹲下时髋角（负是往上收腿）

% 时间设置（和膝盖可以对应着来）
T1 = 3;    % 蹲下用时
T2 = 15;    % 低姿态保持时间
T3 = 3;    % 站起来用时
% 总时长 T1+T2+T3 之后保持站立

% --- 段1：从站立 -> 蹲下 ---
if tau < T1
    u = tau / T1;                      % 0→1
    q = (1-u)*q_stand + u*q_squat;

% --- 段2：保持蹲下姿态 ---
elseif tau < T1 + T2
    q = q_squat;

% --- 段3：从蹲下 -> 站回原位 ---
elseif tau < T1 + T2 + T3
    u = (tau - (T1 + T2)) / T3;
    q = (1-u)*q_squat + u*q_stand;

% --- 结束后：保持站立 ---
else
    q = q_stand;
end
end

== matlab function RobotModel8/RR/MATLAB Function3 ==
  data: brake_en input; tau output; w input
function tau = BrakeTorque(brake_en, w)
%#codegen
% brake_en: 0=不刹车, 1=开始刹车
% w: 轮子角速度 (rad/s)，来自 Revolute Joint 的 Velocity 输出

Kb = 30.0;       % 阻尼系数，越大刹车越狠，可调
tau_max = 150.0; % 最大刹车扭矩限幅
w_eps = 0.05;    % 认为“已经停下”的速度阈值

if brake_en == 0
    tau = 0.0;     % 不刹车
    return;
end

% 速度很小就不再给力，避免抖动
if abs(w) < w_eps
    tau = 0.0;
else
    % 阻尼刹车：扭矩方向与角速度相反
    tau = -Kb * w;
end

% 扭矩限幅
if tau >  tau_max, tau =  tau_max; end
if tau < -tau_max, tau = -tau_max; end
end

== matlab function RobotModel8/FL_climb/MATLAB Function4 ==
  data: t input; q output; mode_cmd input
function q = hip_FL_motion(t, mode_cmd)
%#codegen

Tsw = 102;

% 轮式阶段：髋关节锁在 0
if (mode_cmd == 1) || (t < Tsw)
    q = 0;          % 轮式时锁住髋关节
    return;
end

% 腿式阶段：开始做“先蹲后站”的动作
tau = t - Tsw;      % 本地时间，从切换时刻重新计

% 姿态角（单位：rad）
q_stand = 0;                  % 站立时髋角
q_squat = deg2rad(35);       % 蹲下时髋角（负是往上收腿）

% 时间设置（和膝盖可以对应着来）
T1 = 3;    % 蹲下用时
T2 = 15;    % 低姿态保持时间
T3 = 3;    % 站起来用时
% 总时长 T1+T2+T3 之后保持站立

% --- 段1：从站立 -> 蹲下 ---
if tau < T1
    u = tau / T1;                      % 0→1
    q = (1-u)*q_stand + u*q_squat;

% --- 段2：保持蹲下姿态 ---
elseif tau < T1 + T2
    q = q_squat;

% --- 段3：从蹲下 -> 站回原位 ---
elseif tau < T1 + T2 + T3
    u = (tau - (T1 + T2)) / T3;
    q = (1-u)*q_squat + u*q_stand;

% --- 结束后：保持站立 ---
else
    q = q_stand;
end
end

== matlab function RobotModel8/FR_climb/MATLAB Function1 ==
  data: t input; q output; mode_cmd input
function q = hip_FR_motion(t, mode_cmd)
%#codegen
% --- 右前腿 (Front Right) 髋关节 ---

T_squat_start = 102;
T_climb_start = 130;

% --- 阶段 0 & 1 ---
if (mode_cmd == 1) || (t < T_squat_start); q = 0; return; end
if t < T_climb_start
    tau = t - T_squat_start;
    q_stand = 0; q_squat = deg2rad(35);
    T1 = 3; T2 = 15; T3 = 3;
    if tau < T1; u=tau/T1; q=(1-u)*q_stand+u*q_squat;
    elseif tau < T1+T2; q=q_squat;
    elseif tau < T1+T2+T3; u=(tau-(T1+T2))/T3; q=(1-u)*q_squat+u*q_stand;
    else; q=q_stand; end
    return;
end

% ==========================================
% 阶段 2: 锁轮爬台阶 (130s 开始)
% ==========================================
tau = t - T_climb_start;

q_neutral = 0;
    q_fwd     = deg2rad(-5);
    
    % [130-132] 等待左前腿
    if tau < 4.0
        q = q_neutral;

    % [132-134] 第二步：抬腿迈向前方
    elseif tau < 8.0
        dt = tau - 4.0;
        u = dt / 4.0;
        q = (1-u)*q_neutral + u*q_fwd;
        
    % [134-138] 全身前移 (Body Shift)
    % 同样用力往回拉
    elseif tau < 12.0
        dt = tau - 8.0;
        u = dt / 6.0;
        u_smooth = 0.5 * (1 - cos(u * pi));
        q = (1-u_smooth)*q_fwd + u_smooth*q_neutral;
        
    else
        q = q_neutral;
    end
end

== matlab function RobotModel8/FR_climb/MATLAB Function4 ==
  data: t input; q output; mode_cmd input
function q = knee_FR_motion(t, mode_cmd)
%#codegen
% --- 右前腿 (Front Right) 膝关节 ---

T_squat_start = 102;
T_climb_start = 130;

% --- 阶段 0 & 1 ---
if (mode_cmd == 1) || (t < T_squat_start); q = 0; return; end
if t < T_climb_start
    tau = t - T_squat_start;
    q_stand = 0; q_squat = -deg2rad(70);
    T1 = 3; T2 = 15; T3 = 3;
    if tau < T1; u=tau/T1; q=(1-u)*q_stand+u*q_squat;
    elseif tau < T1+T2; q=q_squat;
    elseif tau < T1+T2+T3; u=(tau-(T1+T2))/T3; q=(1-u)*q_squat+u*q_stand;
    else; q=q_stand; end
    return;
end

% ==========================================
% 阶段 2: 锁轮爬台阶 (130s 开始)
% ==========================================
tau = t - T_climb_start;

q_stand = deg2rad(0);
    q_lift  = deg2rad(-20);

    % [130-132] 等待
    if tau < 4.0
        q = q_stand;
        
    % [132-134] 抬腿迈步
    elseif tau < 8.0
        dt = tau - 4.0;
        u = dt / 4.0;
        lift_scale = sin(u * pi);
        q = q_stand + lift_scale * (q_lift - q_stand);
        
    else
        q = q_stand;
    end
end

== matlab function RobotModel8/RL_climb/MATLAB Function2 ==
  data: t input; q output; mode_cmd input
function q = hip_RL_motion(t, mode_cmd)
%#codegen
% --- 左后腿 (Rear Left) 髋关节 ---
% 策略：锁轮爬行。先蹬地推身体，再收腿上台阶。

T_squat_start = 102;
T_climb_start = 130; 

% --- 阶段 0: 轮式/未开始 ---
if (mode_cmd == 1) || (t < T_squat_start); q = 0; return; end

% --- 阶段 1: 原地蹲起测试 (保持不变) ---
if t < T_climb_start
    tau = t - T_squat_start;
    q_stand = 0; q_squat = deg2rad(35);
    T1 = 3; T2 = 15; T3 = 3;
    if tau < T1; u=tau/T1; q=(1-u)*q_stand+u*q_squat;
    elseif tau < T1+T2; q=q_squat;
    elseif tau < T1+T2+T3; u=(tau-(T1+T2))/T3; q=(1-u)*q_squat+u*q_stand;
    else; q=q_stand;
    end
    return;
end

% ==========================================
% 阶段 2: 锁轮爬台阶 (130s 开始)
% ==========================================
tau = t - T_climb_start;

q_neutral = 0;
    q_push    = deg2rad(15); % 向后蹬的角度
    
    % [130-134] 前腿迈步时，后腿保持不动作为支撑
    if tau < 4.0
        q = q_neutral;
        
    % [134-138] 全身前移 (Body Shift)
    % 关键：前腿在拉，后腿要负责"推"！(从0变到+15)
    elseif tau < 8.0
        dt = tau - 4.0;
        u = dt / 4.0;
        u_smooth = 0.5 * (1 - cos(u * pi));
        q = (1-u_smooth)*q_neutral + u_smooth*q_push;
        
    % [138-140] 第四步：抬腿收回 (Swing Forward)
    % 从"后蹬"状态(+15) 抬起来回到 "中立"(0)
    elseif tau < 10.0
        dt = tau - 8.0;
        u = dt / 2.0;
        q = (1-u)*q_push + u*q_neutral;
        
    else
        q = q_neutral;
    end
end

== matlab function RobotModel8/RL_climb/MATLAB Function3 ==
  data: t input; q output; mode_cmd input
function q = knee_RL_motion(t, mode_cmd)
%#codegen
% --- 左后腿 (Rear Left) 膝关节 ---

T_squat_start = 102;
T_climb_start = 130;

% --- 阶段 0 & 1 (省略，保持不变) ---
if (mode_cmd == 1) || (t < T_squat_start); q = 0; return; end
if t < T_climb_start
    tau = t - T_squat_start;
    q_stand = 0; q_squat = -deg2rad(70);
    T1 = 3; T2 = 15; T3 = 3;
    if tau < T1; u=tau/T1; q=(1-u)*q_stand+u*q_squat;
    elseif tau < T1+T2; q=q_squat;
    elseif tau < T1+T2+T3; u=(tau-(T1+T2))/T3; q=(1-u)*q_squat+u*q_stand;
    else; q=q_stand;
    end
    return;
end

% ==========================================
% 阶段 2: 锁轮爬台阶 (130s 开始)
% ==========================================
tau = t - T_climb_start;

q_stand = deg2rad(0);
    q_lift  = deg2rad(-20);
    
    % [130-138] 支撑 + 推地
    if tau < 8.0
        q = q_stand;
        
    % [138-140] 抬腿收回
    elseif tau < 10.0
        dt = tau - 8.0;
        u = dt / 2.0;
        lift_scale = sin(u * pi);
        q = q_stand + lift_scale * (q_lift - q_stand);
        
    else
        q = q_stand;
    end
end

== matlab function RobotModel8/RR_climb/MATLAB Function2 ==
  data: t input; q output; mode_cmd input
function q = hip_RR_motion(t, mode_cmd)
%#codegen
% --- 右后腿 (Rear Right) 髋关节 ---

T_squat_start = 102;
T_climb_start = 130; 

if (mode_cmd == 1) || (t < T_squat_start); q = 0; return; end
% ... (省略蹲起阶段，请复制上面的) ...
if t < T_climb_start
    tau = t - T_squat_start;
    q_stand = 0; q_squat = deg2rad(35);
    T1 = 3; T2 = 15; T3 = 3;
    if tau < T1; u=tau/T1; q=(1-u)*q_stand+u*q_squat;
    elseif tau < T1+T2; q=q_squat;
    elseif tau < T1+T2+T3; u=(tau-(T1+T2))/T3; q=(1-u)*q_squat+u*q_stand;
    else; q=q_stand;
    end
    return;
end


tau = t - T_climb_start;

q_neutral = 0;
    q_push    = deg2rad(15);
    
    % [130-134] 支撑
    if tau < 4.0
        q = q_neutral;
        
    % [134-138] 推地 (Body Shift)
    elseif tau < 8.0
        dt = tau - 4.0;
        u = dt / 4.0;
        u_smooth = 0.5 * (1 - cos(u * pi));
        q = (1-u_smooth)*q_neutral + u_smooth*q_push;
        
    % [138-140] 等待左后腿收完 (保持推地状态支撑)
    elseif tau < 10.0
        q = q_push;

    % [140-142] 第五步：抬腿收回
    elseif tau < 12.0
        dt = tau - 10.0;
        u = dt / 2.0;
        q = (1-u)*q_push + u*q_neutral;
        
    else
        q = q_neutral;
    end
end

== matlab function RobotModel8/RR_climb/MATLAB Function4 ==
  data: t input; q output; mode_cmd input
function q = knee_RR_motion(t, mode_cmd)
%#codegen
% --- 右后腿 (Rear Right) 膝关节 ---

T_squat_start = 102;
T_climb_start = 130;

if (mode_cmd == 1) || (t < T_squat_start); q = 0; return; end
% ... (省略蹲起阶段) ...
if t < T_climb_start
    tau = t - T_squat_start;
    q_stand = 0; q_squat = -deg2rad(70);
    T1 = 3; T2 = 15; T3 = 3;
    if tau < T1; u=tau/T1; q=(1-u)*q_stand+u*q_squat;
    elseif tau < T1+T2; q=q_squat;
    elseif tau < T1+T2+T3; u=(tau-(T1+T2))/T3; q=(1-u)*q_squat+u*q_stand;
    else; q=q_stand;
    end
    return;
end


tau = t - T_climb_start;

q_stand = deg2rad(0);
    q_lift  = deg2rad(-20);

    % [130-140] 支撑 + 推地
    if tau < 10.0
        q = q_stand;
        
    % [140-142] 抬腿收回
    elseif tau < 12.0
        dt = tau - 10.0;
        u = dt / 2.0;
        lift_scale = sin(u * pi);
        q = q_stand + lift_scale * (q_lift - q_stand);
        
    else
        q = q_stand;
    end
end

== matlab function RobotModel8/RR/MATLAB Function ==
  data: mode_cmd input; alpha input; tau output; q input; dq input; q_cmd input; is_locked output; q_ref output
function [tau, is_locked, q_ref] = LockJointPD(mode_cmd, alpha, q, dq, q_cmd)
%#codegen
% mode_cmd: 0=Walk(folloew q_cmd), 1=Wheel(lock the present angle )
% alpha   : [0,1] flatten faktor(TransferFcnoutput)，0=walk, 1=leg locked
% q,dq    : joint angle/angular velocity
% q_cmd   : walking/standing angle(rad)

Kp = 1200.0;   % start value
Kd =   20.0;
tau_lim = 300.0;

m = uint8(mode_cmd ~= 0);     % uint8(0/1)
a = double(alpha);

persistent q_hold last_mode
if isempty(q_hold),    q_hold    = q;        end   % double
if isempty(last_mode), last_mode = uint8(0); end   % uint8

% step: 0->1 
if (last_mode == uint8(0)) && (m ~= uint8(0))
    q_hold = q;
end
last_mode = m;

% reference angle
q_ref  = a*q_hold + (1-a)*q_cmd;
dq_ref = 0.0;

% PD
tau = Kp*(q_ref - q) + Kd*(dq_ref - dq);

% 
tau = max(min(tau, tau_lim), -tau_lim);

% 
is_locked = (a > 0.5);     % 
end

== matlab function RobotModel8/RL/MATLAB Function4 ==
  data: t input; w output
function w = wheel_speed(t)

%#codegen

% --- 原始参数 ---

Tsw = 105; % 初次开始加速时间

Tacc = 2; % 加速时间 (0 -> V)

V = 100; % 力矩幅值 V

V2 = 20; % 力矩幅值 V2

Tdec_start = 125; % 开始减速 (V -> 0)

Tdec = 3; % 减速时间

Tpause = 5; % 停止后的等待时间

Treacc = 2; % 再次加速时间 (0 -> V2)

% --- 新增参数 (请根据需要调整数值) ---

Thold_V2 = 8; % V2 保持时间 (10秒)

Tdec2 = 3; % 第二次减速时间 (V2 -> 0) [假设为3秒]

Tpause2 = 10; % 第二次停止等待时间 (2秒)

Treacc2 = 2; % 第三次加速时间 (0 -> V2) [假设为2秒]

% --- 为了代码可读性，计算关键时间节点 ---

% 节点 1: V2 第一次加速完成的时间点 (即阶段 6 结束)

T_V2_ready = Tdec_start + Tdec + Tpause + Treacc;

% 节点 2: V2 保持 10秒 结束，开始减速的时间点

T_dec2_start = T_V2_ready + Thold_V2;

% 节点 3: 减速至 0 完成的时间点

T_stop2_start = T_dec2_start + Tdec2;

% 节点 4: 停止 2秒 结束，开始最后加速的时间点

T_last_acc_start = T_stop2_start + Tpause2;

% 节点 5: 最后加速至 V2 完成的时间点

T_final_stable = T_last_acc_start + Treacc2;

% ====================

% 逻辑判断

% ====================

% 阶段 1：未开始

if t < Tsw

w = 0;

% 阶段 2：线性加速 0 -> V

elseif t < Tsw + Tacc

u = (t - Tsw) / Tacc;

w = u * V;

% 阶段 3：保持 V

elseif t < Tdec_start

w = V;

% 阶段 4：线性减速 V -> 0

elseif t < Tdec_start + Tdec

u = (t - Tdec_start) / Tdec;

w = V * (1 - u);

% 阶段 5：停止等待

elseif t < Tdec_start + Tdec + Tpause

w = 0;

% 阶段 6：重新加速 0 -> V2

elseif t < T_V2_ready

u = (t - (Tdec_start + Tdec + Tpause)) / Treacc;

w = u * V2;

% --------------------

% 新增阶段开始

% --------------------

% 阶段 7：保持 V2 (10秒)

elseif t < T_dec2_start

w = V2;

% 阶段 8：再次减速 V2 -> 0

elseif t < T_stop2_start

u = (t - T_dec2_start) / Tdec2;

w = V2 * (1 - u);

% 阶段 9：再次停止等待 (2秒)

elseif t < T_last_acc_start

w = 0;

% 阶段 10：最后加速 0 -> V2

elseif t < T_final_stable

u = (t - T_last_acc_start) / Treacc2;

w = u * V2;

% 阶段 11：永久保持 V2

else

w = V2;

end

== matlab function RobotModel8/RR/MATLAB Function4 ==
  data: t input; w output
function w = wheel_speed(t)
%#codegen

Tsw  = 105;   % 初次开始加速时间
Tacc = 2;     % 加速时间
V    = 100;   % 力矩幅值
Tdec_start = 125;   % 开始减速
Tdec = 3;           % 减速时间

% --------------------
% 阶段 1：未开始
% --------------------
if t < Tsw
    w = 0;

% --------------------
% 阶段 2：线性加速 0→V
% --------------------
elseif t < Tsw + Tacc
    u = (t - Tsw) / Tacc;
    w = u * V;

% --------------------
% 阶段 3：保持 V
% --------------------
elseif t < Tdec_start
    w = V;

% --------------------
% 阶段 4：线性减速 V→0
% --------------------
elseif t < Tdec_start + Tdec
    u = (t - Tdec_start) / Tdec;  % 0→1
    w = V * (1 - u);

else
    w = 0;
end
end

== matlab function RobotModel8/FR/MATLAB Function2 ==
  data: t input; w output
function w = wheel_speed(t)
%#codegen

Tsw  = 105;   % 初次开始加速时间
Tacc = 2;     % 加速时间
V    = 100;   % 力矩幅值
Tdec_start = 125;   % 开始减速
Tdec = 3;           % 减速时间

% --------------------
% 阶段 1：未开始
% --------------------
if t < Tsw
    w = 0;

% --------------------
% 阶段 2：线性加速 0→V
% -------------------
elseif t < Tsw + Tacc
    u = (t - Tsw) / Tacc;
    w = u * V;

% --------------------
% 阶段 3：保持 V
% --------------------
elseif t < Tdec_start
    w = V;

% --------------------
% 阶段 4：线性减速 V→0
% --------------------
elseif t < Tdec_start + Tdec
    u = (t - Tdec_start) / Tdec;  % 0→1
    w = V * (1 - u);

else
    w = 0;
end
end
